simulink model "ext_mode_intro"  (R2017b)
settings: Solver=FixedStepDiscrete  StartTime=0.0  StopTime=inf  FixedStep=1/100  RelTol=1e-3  EnableMultiTasking=on
InitFcn:
  | GainTune = 1;
  | alignTime = floor(398.001 * Ts);
  | EAS2TAS = 1;
  | LatDegInit = 1;
  | LngDegInit = 1;
  | msecVelDelay = 300;
  | msecPosDelay = 300;
  | msecHgtDelay = 420;
  | msecMagDelay = 30;
  | msecTasDelay = 200;
libraries: simulink x9, pixhawk_slib_sensors_actuators x3, simulink_need_slupdate x2
(part 1 of 4)
Description:
  | ext_mode_intro
  | 
  | This model uses ttyS6 on the Pixhawk for the EXT mode serial data exchange.
  | This means the MEX arguments must be set accordingly to use the right COM port.
  | Please check your windows setting (COM8 in this example)
  | COM 6 will be the serial console (ttyACM0)
  | 
  | Note: Baud rate set at 115200
settings Model: SimulationMode=external  Creator=skuznick  LastModifiedBy=tom
settings DataIOCC: LimitDataPoints=on  SaveFormat=Array  SignalLoggingSaveFormat=ModelDataLogs
settings OptimizationCC: DefaultParameterBehavior=Inlined  LifeSpan=1  MaxStackSize=64
settings DebuggingCC: SolverPrmCheckMsg=warning  MultiTaskDSMMsg=warning  MultiTaskCondExecSysMsg=none  AllowSymbolicDim=off  SFUnexpectedBacktrackingDiag=warning  SFNoUnconditionalDefaultTransitionDiag=warning  SFExecutionAtInitializationDiag=none
settings HardwareCC: ProdBitPerPointer=32  ProdBitPerSizeT=32  ProdBitPerPtrDiffT=32  ProdLargestAtomicInteger=Long  ProdLargestAtomicFloat=Double  ProdIntDivRoundTo=Undefined  ProdWordSize=32  ProdHWDeviceType=ARM Compatible->ARM Cortex
settings ModelReferenceCC: PropagateSignalLabelsOutOfModel=off
settings SFSimCC: MATLABDynamicMemAlloc=off
settings RTWCC: SystemTargetFile=ert.tlc  HardwareBoard=Pixhawk PX4  TLCOptions=-aInlineSetEventsForThisBaseRateFcn=TLC_FALSE -aSuppressMultiTaskScheduler=TLC_FALSE -aRateBasedStepFcn=0  TemplateMakefile=ert_default_tmf  GenerateReport=on  Toolchain=Pixhawk Toolchain  IncludeHyperlinkInReport=on  LaunchReport=on  GenerateTraceInfo=on  GenerateTraceReport=on  GenerateTraceReportSl=on  GenerateTraceReportSf=on  GenerateTraceReportEml=on  GenerateCodeMetricsReport=on
settings CodeAppCC: IgnoreCustomStorageClasses=off  StateflowObjectComments=on
settings ERTTargetCC: MultiwordLength=2048  ExtMode=on  ExtModeTransport=1  ExtModeStaticAllocSize=10000  ExtModeMexFile=ext_serial_win32_comm  ExtModeMexArgs=1 '/dev/ttyACM0' 57600 5  ERTCustomFileTemplate=px4_codertarget_file_process.tlc  ConvertIfToSwitch=off  SuppressUnreachableDefaultCases=off
settings ConfigComp: CovMetricSettings=dw  CovHtmlReporting=on  CovSaveCumulativeToWorkspaceVar=on  CovSaveSingleToWorkspaceVar=on  CovExternalEMLEnable=off  CovSFcnEnable=off

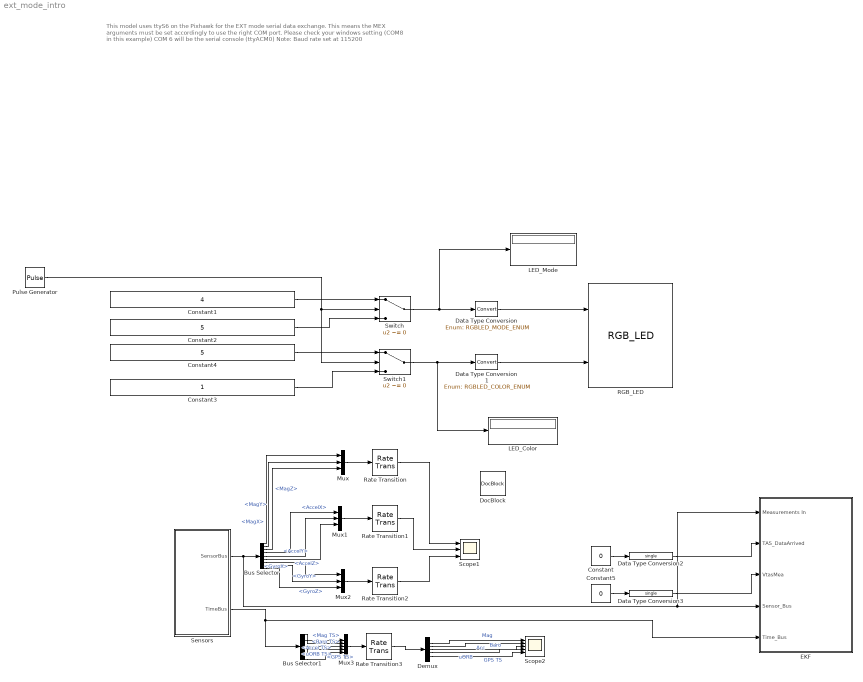
== system ext_mode_intro ==
  note: This model uses ttyS6 on the Pixhawk for the EXT mode serial data exchange.
      | This means the MEX arguments must be set accordingly to use the right COM port.
      | Please check your windows setting (COM8 in this example)
      | COM 6 will be the serial console (ttyACM0)
      |
      | Note: Baud rate set at 115200
  Bus Selector : BusSelector  OutputSignals=MagX,MagY,MagZ,AccelX,AccelY,AccelZ,GyroX,GyroY,GyroZ
  Bus Selector1 : BusSelector  OutputSignals=Mag TS,Accel TS,Baro TS,uORB TS,GPS TS
  Constant : Constant  Value=0  SampleTime=-1
  Constant1 : Constant  Value=4  OutDataTypeStr=int8
  Constant2 : Constant  Value=5  OutDataTypeStr=int8
  Constant3 : Constant  OutDataTypeStr=int8
  Constant4 : Constant  Value=5  OutDataTypeStr=int8
  Constant5 : Constant  Value=0  SampleTime=-1
  Data Type Conversion : DataTypeConversion  OutDataTypeStr=Enum: RGBLED_MODE_ENUM
  Data Type Conversion1 : DataTypeConversion  OutDataTypeStr=Enum: RGBLED_COLOR_ENUM
  Data Type Conversion2 : DataTypeConversion  OutDataTypeStr=single
  Data Type Conversion3 : DataTypeConversion  OutDataTypeStr=single
  Demux : Demux  Outputs=5
  DocBlock : simulink/Model-Wide Utilities/DocBlock  DocumentType=Text
      content=|
      | 24 State Extended Kalman Filter
      |
      | States :
      | 1 ... 4   : Quaternion parameters defining the rotation from local NED tangent frame to XYZ body axes
      | 5 ... 7   : North, East, Down velocity relative to and earth fixed reference point (m)
      | 8 ... 10  : North, East, Down position relative to and earth fixed reference point (m)
      | 11 ... 13 : IMU delta angle bias errors (rad)
      | 14 ... 16 : IMU delta velocity bias errors (m/s)
      | 17,18     : North, East wind velocity (m/s)
      | 19 ... 21 : North, East, Down earth magnetic field (same units as magnetometer output)
      | 22 ... 24 : X, Y, Z Body fixed magnetic field bias - opposite sign to APM offsets (same units as magnetometer output)
      |
      | Time Varying Parameters :
      | IMU delta angles (rad)
      | IMU delta velocity (rad)
      |
      | Observations :
      | North, East, Down velocity (m/s)
      | North, East position (m)
      | Height (m)
      | True Airspeed (m/s) - optional
      | X, Y, Z body fixed magnetic flux measurements (same units as magnetometer output) - optional
      |
      | Note : without compass/magnetometer measurements, the heading alignment cannot be maintained on the ground, so the filter will need to be re-started when flight commences.
      |
      |
      | TO-DO:
      | 1).  Set all signals into a Bus object for cleaner Simulink models.
      | 2).  Incorporate a Complementary filter in the watchdog.
      | 3).  Evaluate EKF model, specificly frequency and parameters.
      | 4).  Tune EKF, Complementary Filter, and controllers for easy angular flight.
      | 5).  Test if all signals are properly connected to the EKF (signs, formats, and representation).
      | 6).  TAS data.
      | 7).  GPS Velocity data.
      | 8).  Include Current measurements to compensate magnetometer.
      | 9).  Include Barometer measurements in EKF.
      | 10). Find out how the reset funtion operates.
  EKF : Subsystem
  LED_Color : Display
  LED_Mode : Display
  Mux : Mux  Inputs=3
  Mux1 : Mux  Inputs=3
  Mux2 : Mux  Inputs=3
  Mux3 : Mux  Inputs=5
  Pulse Generator : DiscretePulseGenerator  PulseType=Time based  Period=6  PulseWidth=50
  RGB_LED : pixhawk_slib_sensors_actuators/RGB_LED
      settings: SourceProductName=Pixhawk Target Blocks
  Rate Transition : RateTransition  InitialCondition=[0; 0; 0]  OutPortSampleTime=0.1
  Rate Transition1 : RateTransition  InitialCondition=[0; 0; 0]  OutPortSampleTime=0.1
  Rate Transition2 : RateTransition  InitialCondition=[0; 0; 0]  OutPortSampleTime=0.1
  Rate Transition3 : RateTransition  InitialCondition=[0; 0; 0; 0; 0]  OutPortSampleTime=0.1
  Scope1 : Scope  NumInputPorts=3
  Scope2 : Scope  NumInputPorts=5
  "Sensors " : Subsystem
  Switch : Switch  Criteria=u2 ~= 0  Threshold=1500
  Switch1 : Switch  Criteria=u2 ~= 0  Threshold=1500
  wires:
  Switch/1 -> LED_Mode/1, Data Type Conversion/1
  Switch1/1 -> LED_Color/1, Data Type Conversion1/1
  Constant1/1 -> Switch/1
  Constant2/1 -> Switch/3
  Constant4/1 -> Switch1/1
  Constant3/1 -> Switch1/3
  Pulse Generator/1 -> Switch1/2, Switch/2
  Data Type Conversion/1 -> RGB_LED/1
  Data Type Conversion1/1 -> RGB_LED/2
  Bus Selector/3 -> Mux/3  "<MagZ>"
  Bus Selector/2 -> Mux/2  "<MagY>"
  Bus Selector/1 -> Mux/1  "<MagX>"
  Bus Selector/6 -> Mux1/3  "<AccelZ>"
  Bus Selector/5 -> Mux1/2  "<AccelY>"
  Bus Selector/4 -> Mux1/1  "<AccelX>"
  Bus Selector/7 -> Mux2/1  "<GyroX>"
  Bus Selector/8 -> Mux2/2  "<GyroY>"
  Bus Selector/9 -> Mux2/3  "<GyroZ>"
  Mux/1 -> Rate Transition/1
  Mux1/1 -> Rate Transition1/1
  Mux2/1 -> Rate Transition2/1
  Rate Transition/1 -> Scope1/1
  Rate Transition1/1 -> Scope1/2
  Rate Transition2/1 -> Scope1/3
  Constant/1 -> Data Type Conversion2/1
  Data Type Conversion2/1 -> EKF/2(TAS_DataArrived)
  Constant5/1 -> Data Type Conversion3/1
  Data Type Conversion3/1 -> EKF/3(VtasMea)
  "Sensors "/1(SensorBus) -> EKF/4(Sensor_Bus), EKF/1(Measurements In), Bus Selector/1
  Bus Selector1/1 -> Mux3/1  "<Mag TS>"
  Bus Selector1/2 -> Mux3/2  "<Accel TS>"
  Bus Selector1/3 -> Mux3/3  "<Baro TS>"
  Bus Selector1/4 -> Mux3/4  "<uORB TS>"
  Mux3/1 -> Rate Transition3/1
  Rate Transition3/1 -> Demux/1
  Demux/1 -> Scope2/1  "Mag"
  Demux/2 -> Scope2/2  "Acc"
  Demux/3 -> Scope2/3  "Baro"
  Demux/4 -> Scope2/4  "uORB"
  "Sensors "/2(TimeBus) -> EKF/5(Time_Bus), Bus Selector1/1
  Bus Selector1/5 -> Mux3/5  "<GPS TS>"
  Demux/5 -> Scope2/5  "GPS TS"

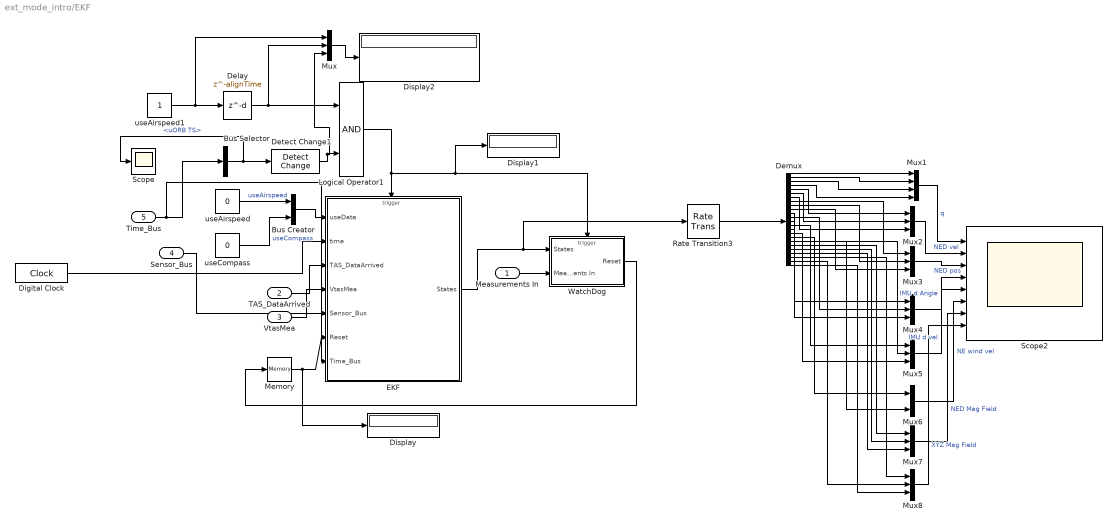
== system ext_mode_intro/EKF ==
  Measurements In : Inport
  TAS_DataArrived : Inport  Port=2
  VtasMea : Inport  Port=3
  Sensor_Bus : Inport  Port=4
  Time_Bus : Inport  Port=5
  Bus Creator : BusCreator  Inputs=2
  Bus Selector : BusSelector  OutputSignals=uORB TS
  Delay : Delay  DelayLength=alignTime  InitialCondition=0
  Demux : Demux  Outputs=24
  Detect Change1 : simulink/Logic and Bit Operations/Detect Change  vinit=0  InputProcessing=Inherited  OutDataTypeStr=boolean
  Digital Clock : DigitalClock  SampleTime=-1
  Display : Display
  Display1 : Display
  Display2 : Display
  EKF : Subsystem
  Logical Operator1 : Logic  AllPortsSameDT=off  OutDataTypeStr=boolean
  Memory : Memory  InheritSampleTime=on
  Mux{,2..5,7..8} (7 alike) : Mux  Inputs=3
  Mux1 : Mux
  Mux6 : Mux  Inputs=2
  Rate Transition3 : RateTransition  InitialCondition=zeros(24,1)  OutPortSampleTime=0.1
  Scope : Scope
  Scope2 : Scope  NumInputPorts=8
  WatchDog : Subsystem  TreatAsAtomicUnit=on
  useAirspeed : Constant  Value=0  OutDataTypeStr=boolean  SampleTime=-1
  useAirspeed1 : Constant  OutDataTypeStr=boolean  SampleTime=-1
  useCompass : Constant  Value=0  OutDataTypeStr=boolean  SampleTime=-1
  wires:
  Measurements In/1 -> WatchDog/2(Measurements In)
  useAirspeed/1 -> Bus Creator/1  "useAirspeed"
  useCompass/1 -> Bus Creator/2  "useCompass"
  EKF/1(States) -> Rate Transition3/1, WatchDog/1(States)
  Logical Operator1/1 -> Display1/1, WatchDog/Trigger, EKF/Trigger
  Memory/1 -> Display/1, EKF/6(Reset)
  WatchDog/1(Reset) -> Memory/1
  Detect Change1/1 -> Mux/3, Logical Operator1/2
  Delay/1 -> Mux/2, Logical Operator1/1
  TAS_DataArrived/1 -> EKF/3(TAS_DataArrived)
  VtasMea/1 -> EKF/4(VtasMea)
  Sensor_Bus/1 -> EKF/5(Sensor_Bus)
  Bus Selector/1 -> Scope/1, Detect Change1/1  "<uORB TS>"
  Bus Creator/1 -> EKF/1(useData)
  useAirspeed1/1 -> Mux/1, Delay/1
  Digital Clock/1 -> EKF/2(time)
  Mux/1 -> Display2/1
  Time_Bus/1 -> EKF/7(Time_Bus), Bus Selector/1
  Rate Transition3/1 -> Demux/1
  Demux/1 -> Mux1/1
  Demux/2 -> Mux1/2
  Demux/3 -> Mux1/3
  Demux/4 -> Mux1/4
  Mux1/1 -> Scope2/1  "q"
  Demux/5 -> Mux2/1
  Demux/6 -> Mux2/2
  Demux/7 -> Mux2/3
  Mux2/1 -> Scope2/2  "NED vel"
  Demux/8 -> Mux3/1
  Demux/9 -> Mux3/2
  Demux/10 -> Mux3/3
  Mux3/1 -> Scope2/3  "NED pos"
  Demux/11 -> Mux4/1
  Demux/12 -> Mux4/2
  Demux/13 -> Mux4/3
  Mux4/1 -> Scope2/4  "IMU d Angle"
  Demux/14 -> Mux5/1
  Demux/15 -> Mux5/2
  Demux/16 -> Mux5/3
  Mux5/1 -> Scope2/5  "IMU d vel"
  Demux/17 -> Mux6/1
  Demux/18 -> Mux6/2
  Mux6/1 -> Scope2/6  "NE wind vel"
  Demux/19 -> Mux7/1
  Demux/20 -> Mux7/2
  Demux/21 -> Mux7/3
  Demux/22 -> Mux8/1
  Demux/23 -> Mux8/2
  Demux/24 -> Mux8/3
  Mux7/1 -> Scope2/7  "NED Mag Field"
  Mux8/1 -> Scope2/8  "XYZ Mag Field"

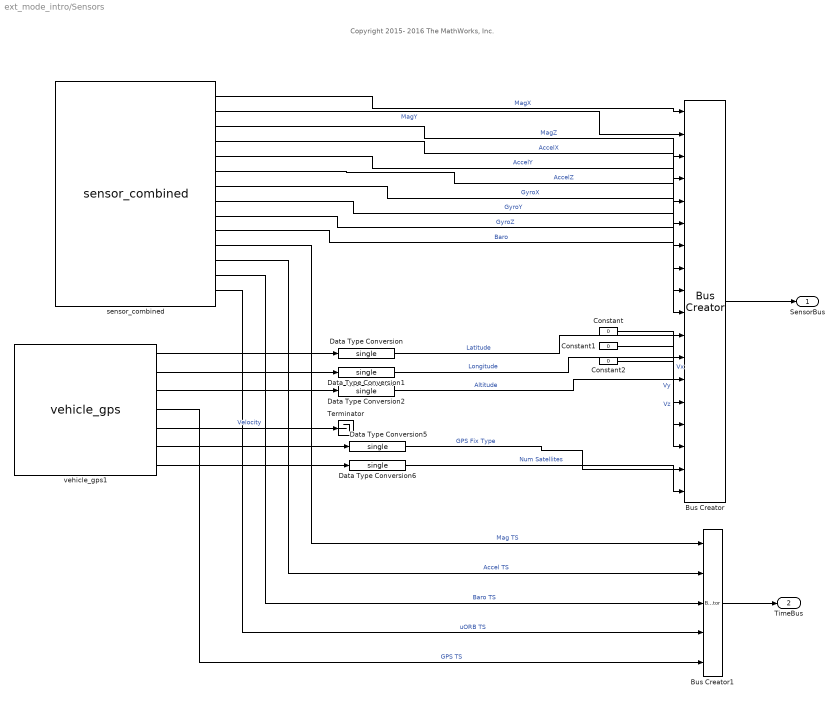
== system ext_mode_intro/Sensors  ==
  note: Copyright 2015- 2016 The MathWorks, Inc.
  Bus Creator : BusCreator  Inputs=18
  Bus Creator1 : BusCreator  Inputs=5
  Constant : Constant  Value=0  OutDataTypeStr=single  SampleTime=-1
  Constant1 : Constant  Value=0  OutDataTypeStr=single  SampleTime=-1
  Constant2 : Constant  Value=0  OutDataTypeStr=single  SampleTime=-1
  Data Type Conversion{,1..2,5..6} (5 alike) : DataTypeConversion  OutDataTypeStr=single
  Terminator : Terminator
  sensor_combined : pixhawk_slib_sensors_actuators/sensor_combined  Description=|  sampletime=-1  show_mag=on  show_acc=on  show_gyro=on  show_baro=on  show_ts=on
      | Sensor Combined Block
      | 
      | This block enables access to the various sensors available on the px4fmu-v2 hardware.  
      | The user can use these signals in the Simulink control model.  
      | The sample time needs to be provided in the mask dialog.  
      | Optional output ports can also be selected.  
      | Refer to the sample model: px4demo_attitude_control.slx
      | 
      | Signal definitions: 
      | Magnetometer (x,y,z) - single values – Magnetic field in NED body frame, in Gauss 
      | Accelerometer (x,y,z) - single values – Acceleration in NED body frame, in m/s^2 
      | Gyroscope (p,q,r) - single values – Angular velocity in radians per second 
      | Barometer (Altitude) - single value – Barometric pressure, already temperature compensated (millibars) 
      | RunTime (timestamp) - double value – Timestamp in microseconds since boot, from gyro 
      |   
      | The sensor_combined block needs to have the px4io service running on the PX4 hardware in order to get valid signal values.
      settings: SourceProductName=Pixhawk Target Blocks
  vehicle_gps1 : pixhawk_slib_sensors_actuators/vehicle_gps  sampletime=-1  show_alt=on  show_ts_gps=on  show_vel=on  show_fixtype=on  show_numsat=on
      settings: SourceProductName=Pixhawk Target Blocks
  SensorBus : Outport
  TimeBus : Outport  Port=2
  wires:
  sensor_combined/1 -> Bus Creator/1  "MagX"
  sensor_combined/2 -> Bus Creator/2  "MagY"
  sensor_combined/3 -> Bus Creator/3  "MagZ"
  sensor_combined/7 -> Bus Creator/7  "GyroX"
  sensor_combined/8 -> Bus Creator/8  "GyroY"
  sensor_combined/9 -> Bus Creator/9  "GyroZ"
  sensor_combined/4 -> Bus Creator/4  "AccelX"
  sensor_combined/5 -> Bus Creator/5  "AccelY"
  sensor_combined/6 -> Bus Creator/6  "AccelZ"
  sensor_combined/10 -> Bus Creator/10  "Baro"
  vehicle_gps1/1 -> Data Type Conversion/1
  vehicle_gps1/2 -> Data Type Conversion1/1
  vehicle_gps1/3 -> Data Type Conversion2/1
  vehicle_gps1/6 -> Data Type Conversion5/1
  vehicle_gps1/7 -> Data Type Conversion6/1
  Bus Creator/1 -> SensorBus/1
  vehicle_gps1/5 -> Terminator/1  "Velocity"
  Data Type Conversion/1 -> Bus Creator/11  "Latitude"
  Data Type Conversion1/1 -> Bus Creator/12  "Longitude"
  Data Type Conversion2/1 -> Bus Creator/13  "Altitude"
  Data Type Conversion5/1 -> Bus Creator/17  "GPS Fix Type"
  Data Type Conversion6/1 -> Bus Creator/18  "Num Satellites"
  Constant/1 -> Bus Creator/14  "Vx"
  Constant1/1 -> Bus Creator/15  "Vy"
  Constant2/1 -> Bus Creator/16  "Vz"
  sensor_combined/14 -> Bus Creator1/4  "uORB TS"
  sensor_combined/13 -> Bus Creator1/3  "Baro TS"
  sensor_combined/12 -> Bus Creator1/2  "Accel TS"
  sensor_combined/11 -> Bus Creator1/1  "Mag TS"
  vehicle_gps1/4 -> Bus Creator1/5  "GPS TS"
  Bus Creator1/1 -> TimeBus/1

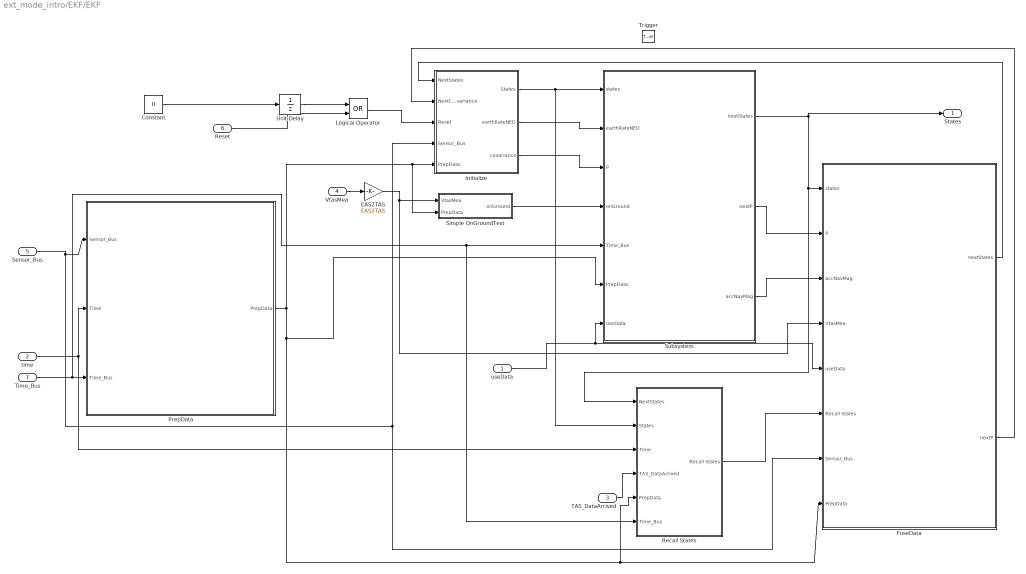
== system ext_mode_intro/EKF/EKF ==
  useData : Inport  OutDataTypeStr=boolean
  time : Inport  Port=2  OutDataTypeStr=double  PortDimensions=1
  TAS_DataArrived : Inport  Port=3
  VtasMea : Inport  Port=4
  Sensor_Bus : Inport  Port=5
  Reset : Inport  Port=6  OutDataTypeStr=boolean  PortDimensions=1
  Time_Bus : Inport  Port=7  OutDataTypeStr=double
  Trigger : TriggerPort  VariantControl=(inherit)  PortDimensions=1
  Constant : Constant  Value=0  OutDataTypeStr=boolean  SampleTime=-1
  EAS2TAS : Gain  Gain=EAS2TAS
  FuseData : Subsystem
  Initialize : Subsystem
  Logical Operator : Logic  Operator=OR  AllPortsSameDT=off  OutDataTypeStr=boolean
  PrepData : Subsystem
  Recall States : Subsystem
  Simple OnGroundTest : Subsystem  TreatAsAtomicUnit=on
  Subsystem : Subsystem
  Unit Delay : UnitDelay  InitialCondition=1  SampleTime=-1
  States : Outport  OutDataTypeStr=single  PortDimensions=24
  wires:
  time/1 -> Recall States/3(Time), PrepData/2(Time)
  Unit Delay/1 -> Logical Operator/1
  Logical Operator/1 -> Initialize/3(Reset)
  Initialize/1(States) -> Subsystem/1(states), Recall States/2(States)
  Reset/1 -> Logical Operator/2
  VtasMea/1 -> EAS2TAS/1
  Sensor_Bus/1 -> PrepData/1(Sensor_Bus), FuseData/7(Sensor_Bus), Initialize/4(Sensor_Bus)
  Constant/1 -> Unit Delay/1
  EAS2TAS/1 -> FuseData/4(VtasMea), Simple OnGroundTest/1(VtasMea)
  Subsystem/1(nextStates) -> States/1, Recall States/1(NextStates), FuseData/1(states)
  Initialize/2(earthRateNED) -> Subsystem/2(earthRateNED)
  Initialize/3(covariance) -> Subsystem/3(P)
  Simple OnGroundTest/1(onGround) -> Subsystem/4(onGround)
  Subsystem/2(nextP) -> FuseData/2(P)
  Subsystem/3(accNavMag) -> FuseData/3(accNavMag)
  FuseData/1(nextStates) -> Initialize/1(NextStates)
  FuseData/2(nextP) -> Initialize/2(NextCovariance)
  TAS_DataArrived/1 -> Recall States/4(TAS_DataArrived)
  useData/1 -> Subsystem/7(useData), FuseData/5(useData)
  Recall States/1(Recall States) -> FuseData/6(Recall States)
  PrepData/1(PrepData) -> Recall States/5(PrepData), FuseData/8(PrepData), Subsystem/6(PrepData), Simple OnGroundTest/2(PrepData), Initialize/5(PrepData)
  Time_Bus/1 -> Recall States/6(Time_Bus), Subsystem/5(Time_Bus), PrepData/3(Time_Bus)

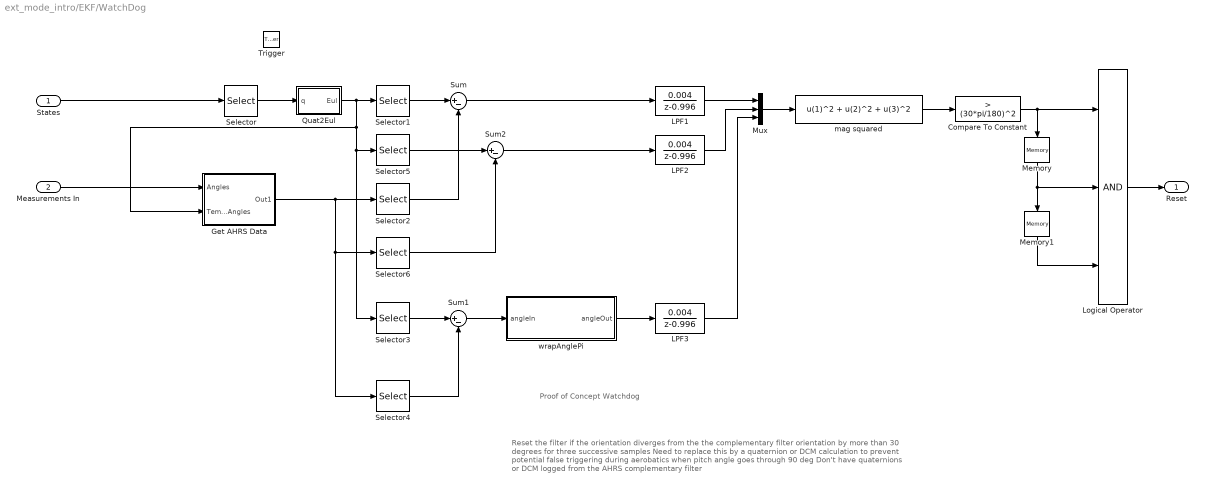
== system ext_mode_intro/EKF/WatchDog ==
  note: Reset the filter if the orientation diverges from the the complementary filter orientation  by more than 30 degrees for three successive samples
      | Need to replace this by a quaternion or DCM calculation to prevent potential false triggering during aerobatics when pitch angle goes through 90 deg
      | Don't have quaternions or DCM logged from the AHRS complementary filter
  note: Proof of Concept Watchdog
  States : Inport
  Measurements In : Inport  Port=2
  Trigger : TriggerPort  VariantControl=(inherit)  PortDimensions=1
  Compare To Constant : simulink/Logic and Bit Operations/Compare To Constant  relop=>  const=(30*pi/180)^2  OutDataTypeStr=boolean
  Get AHRS Data : Subsystem
  LPF1 : DiscreteTransferFcn  Numerator=0.004  Denominator=[1 -0.996]
  LPF2 : DiscreteTransferFcn  Numerator=0.004  Denominator=[1 -0.996]
  LPF3 : DiscreteTransferFcn  Numerator=0.004  Denominator=[1 -0.996]
  Logical Operator : Logic  Inputs=3  AllPortsSameDT=off  OutDataTypeStr=boolean
  Memory : Memory  InheritSampleTime=on
  Memory1 : Memory  InheritSampleTime=on
  Mux : Mux  Inputs=3
  Quat2Eul : Subsystem
  Selector : Selector  InputPortWidth=24  IndexOptions=Index vector (dialog)  Indices=[1:4]  OutputSizes=1
  Selector1 : Selector  InputPortWidth=3  IndexOptions=Index vector (dialog)  Indices=1  OutputSizes=1
  Selector2 : Selector  InputPortWidth=3  IndexOptions=Index vector (dialog)  Indices=1  OutputSizes=1
  Selector3 : Selector  InputPortWidth=3  IndexOptions=Index vector (dialog)  Indices=3  OutputSizes=1
  Selector4 : Selector  InputPortWidth=3  IndexOptions=Index vector (dialog)  Indices=3  OutputSizes=1
  Selector5 : Selector  InputPortWidth=3  IndexOptions=Index vector (dialog)  Indices=2  OutputSizes=1
  Selector6 : Selector  InputPortWidth=3  IndexOptions=Index vector (dialog)  Indices=2  OutputSizes=1
  Sum : Sum  Inputs=|+-
  Sum1 : Sum  Inputs=|+-
  Sum2 : Sum  Inputs=|+-
  mag squared : Fcn  Expr=u(1)^2 + u(2)^2 + u(3)^2
  wrapAnglePi : MATLAB Function  TreatAsAtomicUnit=on
  Reset : Outport  OutDataTypeStr=boolean  PortDimensions=1
  wires:
  Selector/1 -> Quat2Eul/1(q)
  States/1 -> Selector/1
  Quat2Eul/1(Eul) -> Selector1/1, Get AHRS Data/2(Temp Angles), Selector3/1, Selector5/1
  Get AHRS Data/1(Out1) -> Selector2/1, Selector4/1, Selector6/1
  Selector3/1 -> Sum1/1
  Selector4/1 -> Sum1/2
  Sum1/1 -> wrapAnglePi/1(angleIn)
  Sum/1 -> LPF1/1
  wrapAnglePi/1(angleOut) -> LPF3/1
  Mux/1 -> mag squared/1
  mag squared/1 -> Compare To Constant/1
  Compare To Constant/1 -> Logical Operator/1, Memory/1
  Logical Operator/1 -> Reset/1
  Memory/1 -> Logical Operator/2, Memory1/1
  Memory1/1 -> Logical Operator/3
  Selector1/1 -> Sum/1
  Selector2/1 -> Sum/2
  Selector5/1 -> Sum2/1
  Selector6/1 -> Sum2/2
  Sum2/1 -> LPF2/1
  LPF1/1 -> Mux/1
  LPF2/1 -> Mux/2
  LPF3/1 -> Mux/3
  Measurements In/1 -> Get AHRS Data/1(Angles)

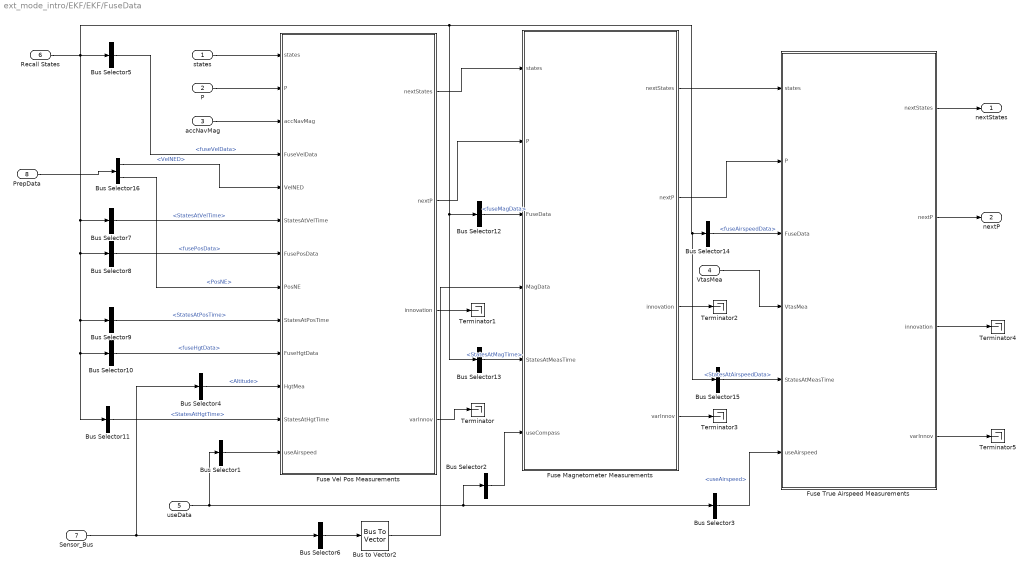
== system ext_mode_intro/EKF/EKF/FuseData ==
  states : Inport
  P : Inport  Port=2
  accNavMag : Inport  Port=3
  VtasMea : Inport  Port=4
  useData : Inport  Port=5
  Recall States : Inport  Port=6
  Sensor_Bus : Inport  Port=7
  PrepData : Inport  Port=8
  Bus Selector1 : BusSelector  OutputSignals=useAirspeed  OutputAsBus=on
  Bus Selector10 : BusSelector  OutputSignals=fuseHgtData
  Bus Selector11 : BusSelector  OutputSignals=StatesAtHgtTime
  Bus Selector12 : BusSelector  OutputSignals=fuseMagData
  Bus Selector13 : BusSelector  OutputSignals=StatesAtMagTime
  Bus Selector14 : BusSelector  OutputSignals=fuseAirspeedData
  Bus Selector15 : BusSelector  OutputSignals=StatesAtAirspeedData
  Bus Selector16 : BusSelector  OutputSignals=VelNED,PosNE
  Bus Selector2 : BusSelector  OutputSignals=useCompass  OutputAsBus=on
  Bus Selector3 : BusSelector  OutputSignals=useAirspeed
  Bus Selector4 : BusSelector  OutputSignals=Altitude
  Bus Selector5 : BusSelector  OutputSignals=fuseVelData
  Bus Selector6 : BusSelector  OutputSignals=MagX,MagY,MagZ  OutputAsBus=on
  Bus Selector7 : BusSelector  OutputSignals=StatesAtVelTime
  Bus Selector8 : BusSelector  OutputSignals=fusePosData
  Bus Selector9 : BusSelector  OutputSignals=StatesAtPosTime
  Bus to Vector2 : BusToVector
  Fuse Magnetometer Measurements : MATLAB Function  TreatAsAtomicUnit=on
  Fuse True Airspeed Measurements : MATLAB Function  TreatAsAtomicUnit=on
  Fuse Vel Pos Measurements : MATLAB Function  TreatAsAtomicUnit=on
  Terminator{,1..5} (6 alike) : Terminator
  nextStates : Outport
  nextP : Outport  Port=2
  wires:
  Bus Selector2/1 -> Fuse Magnetometer Measurements/6(useCompass)
  accNavMag/1 -> Fuse Vel Pos Measurements/3(accNavMag)
  Bus Selector16/1 -> Fuse Vel Pos Measurements/5(VelNED)  "<VelNED>"
  Bus Selector16/2 -> Fuse Vel Pos Measurements/8(PosNE)  "<PosNE>"
  VtasMea/1 -> Fuse True Airspeed Measurements/4(VtasMea)
  Bus Selector1/1 -> Fuse Vel Pos Measurements/13(useAirspeed)
  states/1 -> Fuse Vel Pos Measurements/1(states)
  Bus to Vector2/1 -> Fuse Magnetometer Measurements/4(MagData)
  Fuse Vel Pos Measurements/2(nextP) -> Fuse Magnetometer Measurements/2(P)
  Bus Selector4/1 -> Fuse Vel Pos Measurements/11(HgtMea)  "<Altitude>"
  Fuse Magnetometer Measurements/2(nextP) -> Fuse True Airspeed Measurements/2(P)
  Bus Selector8/1 -> Fuse Vel Pos Measurements/7(FusePosData)  "<fusePosData>"
  Bus Selector5/1 -> Fuse Vel Pos Measurements/4(FuseVelData)  "<fuseVelData>"
  Bus Selector13/1 -> Fuse Magnetometer Measurements/5(StatesAtMeasTime)  "<StatesAtMagTime>"
  Bus Selector7/1 -> Fuse Vel Pos Measurements/6(StatesAtVelTime)  "<StatesAtVelTime>"
  Bus Selector12/1 -> Fuse Magnetometer Measurements/3(FuseData)  "<fuseMagData>"
  Recall States/1 -> Bus Selector13/1, Bus Selector12/1, Bus Selector15/1, Bus Selector14/1, Bus Selector11/1, Bus Selector10/1, Bus Selector9/1, Bus Selector8/1, Bus Selector7/1, Bus Selector5/1
  Bus Selector10/1 -> Fuse Vel Pos Measurements/10(FuseHgtData)  "<fuseHgtData>"
  Fuse Vel Pos Measurements/1(nextStates) -> Fuse Magnetometer Measurements/1(states)
  Fuse True Airspeed Measurements/1(nextStates) -> nextStates/1
  Bus Selector9/1 -> Fuse Vel Pos Measurements/9(StatesAtPosTime)  "<StatesAtPosTime>"
  Fuse True Airspeed Measurements/2(nextP) -> nextP/1
  Fuse Magnetometer Measurements/1(nextStates) -> Fuse True Airspeed Measurements/1(states)
  Bus Selector11/1 -> Fuse Vel Pos Measurements/12(StatesAtHgtTime)  "<StatesAtHgtTime>"
  Bus Selector15/1 -> Fuse True Airspeed Measurements/5(StatesAtMeasTime)  "<StatesAtAirspeedData>"
  Fuse Vel Pos Measurements/3(innovation) -> Terminator1/1
  Fuse Vel Pos Measurements/4(varInnov) -> Terminator/1
  Fuse Magnetometer Measurements/3(innovation) -> Terminator2/1
  Fuse Magnetometer Measurements/4(varInnov) -> Terminator3/1
  Fuse True Airspeed Measurements/3(innovation) -> Terminator4/1
  P/1 -> Fuse Vel Pos Measurements/2(P)
  Fuse True Airspeed Measurements/4(varInnov) -> Terminator5/1
  Bus Selector6/1 -> Bus to Vector2/1
  useData/1 -> Bus Selector1/1, Bus Selector2/1, Bus Selector3/1
  Bus Selector3/1 -> Fuse True Airspeed Measurements/6(useAirspeed)  "<useAirspeed>"
  Sensor_Bus/1 -> Bus Selector6/1, Bus Selector4/1
  Bus Selector14/1 -> Fuse True Airspeed Measurements/3(FuseData)  "<fuseAirspeedData>"
  PrepData/1 -> Bus Selector16/1

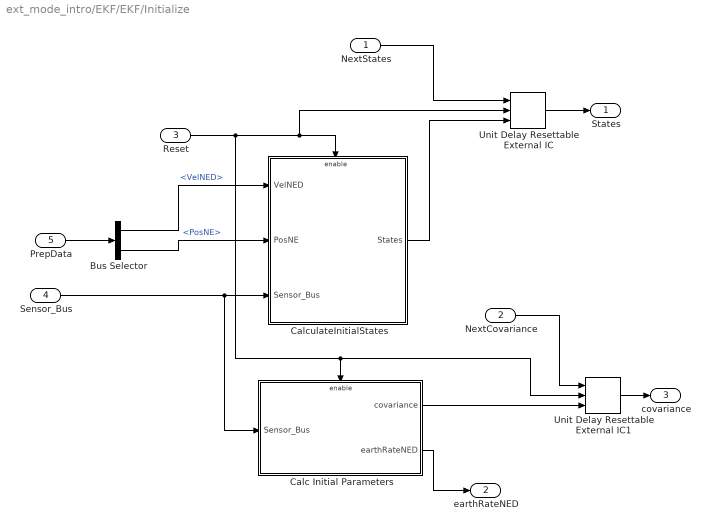
== system ext_mode_intro/EKF/EKF/Initialize ==
  NextStates : Inport
  NextCovariance : Inport  Port=2
  Reset : Inport  Port=3
  Sensor_Bus : Inport  Port=4
  PrepData : Inport  Port=5
  Bus Selector : BusSelector  OutputSignals=VelNED,PosNE
  Calc Initial Parameters : Subsystem
  CalculateInitialStates : Subsystem  TreatAsAtomicUnit=on
  Unit Delay Resettable External IC : simulink_need_slupdate/Unit Delay Resettable External IC  tsamp=-1
      settings: SourceProductName=Simulink  SourceProductBaseCode=SL
  Unit Delay Resettable External IC1 : simulink_need_slupdate/Unit Delay Resettable External IC  tsamp=-1
      settings: SourceProductName=Simulink  SourceProductBaseCode=SL
  States : Outport
  earthRateNED : Outport  Port=2
  covariance : Outport  Port=3
  wires:
  Sensor_Bus/1 -> Calc Initial Parameters/1(Sensor_Bus), CalculateInitialStates/3(Sensor_Bus)
  Bus Selector/1 -> CalculateInitialStates/1(VelNED)  "<VelNED>"
  Reset/1 -> Unit Delay Resettable External IC1/2, Calc Initial Parameters/Enable, Unit Delay Resettable External IC/2, CalculateInitialStates/Enable
  Bus Selector/2 -> CalculateInitialStates/2(PosNE)  "<PosNE>"
  CalculateInitialStates/1(States) -> Unit Delay Resettable External IC/3
  Unit Delay Resettable External IC/1 -> States/1
  NextStates/1 -> Unit Delay Resettable External IC/1
  Calc Initial Parameters/2(earthRateNED) -> earthRateNED/1
  Calc Initial Parameters/1(covariance) -> Unit Delay Resettable External IC1/3
  NextCovariance/1 -> Unit Delay Resettable External IC1/1
  Unit Delay Resettable External IC1/1 -> covariance/1
  PrepData/1 -> Bus Selector/1

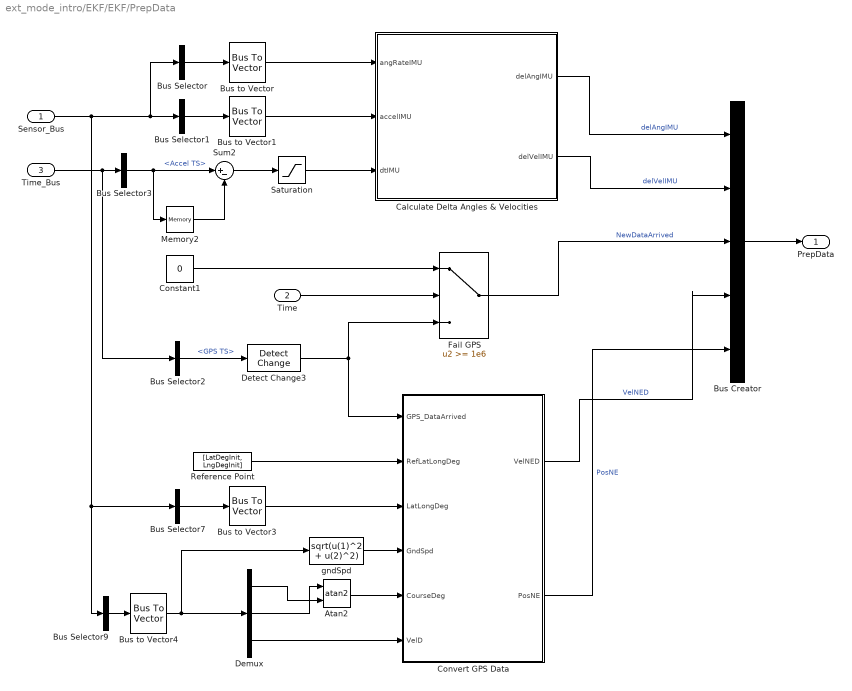
== system ext_mode_intro/EKF/EKF/PrepData ==
  Sensor_Bus : Inport
  Time : Inport  Port=2
  Time_Bus : Inport  Port=3
  Atan2 : Trigonometry  Operator=atan2
  Bus Creator : BusCreator  Inputs=5
  Bus Selector : BusSelector  OutputSignals=GyroX,GyroY,GyroZ  OutputAsBus=on
  Bus Selector1 : BusSelector  OutputSignals=AccelX,AccelY,AccelZ  OutputAsBus=on
  Bus Selector2 : BusSelector  OutputSignals=GPS TS
  Bus Selector3 : BusSelector  OutputSignals=Accel TS
  Bus Selector7 : BusSelector  OutputSignals=Latitude,Longitude  OutputAsBus=on
  Bus Selector9 : BusSelector  OutputSignals=Vx,Vy,Vz  OutputAsBus=on
  Bus to Vector{,1,3..4} (4 alike) : BusToVector
  Calculate Delta Angles & Velocities : MATLAB Function  TreatAsAtomicUnit=on
  Constant1 : Constant  Value=0  OutDataTypeStr=boolean
  Convert GPS Data : MATLAB Function  TreatAsAtomicUnit=on
  Demux : Demux  Outputs=3
  Detect Change3 : simulink/Logic and Bit Operations/Detect Change  vinit=0  InputProcessing=Inherited  OutDataTypeStr=boolean
  Fail GPS : Switch  Threshold=1e6
  Memory2 : Memory  InheritSampleTime=on
  Reference Point : Constant  Value=[LatDegInit, LngDegInit]  OutDataTypeStr=single
  Saturation : Saturate  UpperLimit=0.04  LowerLimit=0
  Sum2 : Sum  Inputs=|+-  AccumDataTypeStr=single
  gndSpd : Fcn  Expr=sqrt(u(1)^2 + u(2)^2)
  PrepData : Outport
  wires:
  Fail GPS/1 -> Bus Creator/3  "NewDataArrived"
  Detect Change3/1 -> Convert GPS Data/1(GPS_DataArrived), Fail GPS/3
  Saturation/1 -> Calculate Delta Angles & Velocities/3(dtIMU)
  Calculate Delta Angles & Velocities/2(delVelIMU) -> Bus Creator/2  "delVelIMU"
  Calculate Delta Angles & Velocities/1(delAngIMU) -> Bus Creator/1  "delAngIMU"
  Convert GPS Data/1(VelNED) -> Bus Creator/4  "VelNED"
  Convert GPS Data/2(PosNE) -> Bus Creator/5  "PosNE"
  Bus to Vector1/1 -> Calculate Delta Angles & Velocities/2(accelIMU)
  Constant1/1 -> Fail GPS/1
  Reference Point/1 -> Convert GPS Data/2(RefLatLongDeg)
  gndSpd/1 -> Convert GPS Data/4(GndSpd)
  Atan2/1 -> Convert GPS Data/5(CourseDeg)
  Demux/3 -> Convert GPS Data/6(VelD)
  Time/1 -> Fail GPS/2
  Bus to Vector3/1 -> Convert GPS Data/3(LatLongDeg)
  Bus Selector/1 -> Bus to Vector/1
  Bus to Vector/1 -> Calculate Delta Angles & Velocities/1(angRateIMU)
  Bus Selector1/1 -> Bus to Vector1/1
  Bus Selector9/1 -> Bus to Vector4/1
  Bus to Vector4/1 -> gndSpd/1, Demux/1
  Demux/1 -> Atan2/2
  Demux/2 -> Atan2/1
  Bus Selector7/1 -> Bus to Vector3/1
  Sensor_Bus/1 -> Bus Selector/1, Bus Selector1/1, Bus Selector7/1, Bus Selector9/1
  Bus Selector2/1 -> Detect Change3/1  "<GPS TS>"
  Memory2/1 -> Sum2/2
  Bus Selector3/1 -> Sum2/1, Memory2/1  "<Accel TS>"
  Sum2/1 -> Saturation/1
  Bus Creator/1 -> PrepData/1
  Time_Bus/1 -> Bus Selector2/1, Bus Selector3/1

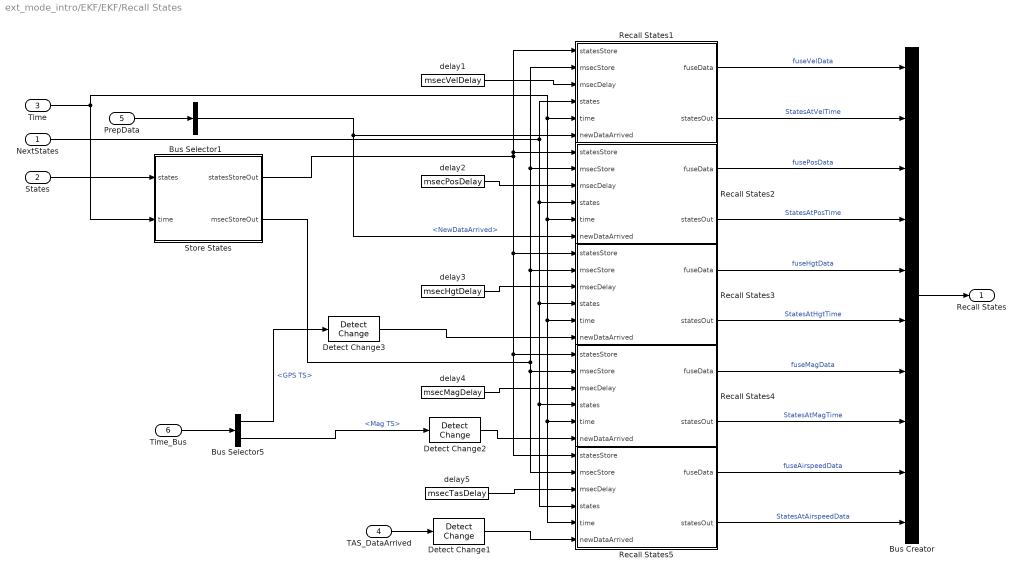
== system ext_mode_intro/EKF/EKF/Recall States ==
  NextStates : Inport
  States : Inport  Port=2
  Time : Inport  Port=3
  TAS_DataArrived : Inport  Port=4
  PrepData : Inport  Port=5
  Time_Bus : Inport  Port=6
  Bus Creator : BusCreator  Inputs=10
  Bus Selector1 : BusSelector  OutputSignals=NewDataArrived
  Bus Selector5 : BusSelector  OutputSignals=GPS TS,Mag TS
  Detect Change1 : simulink/Logic and Bit Operations/Detect Change  vinit=0  InputProcessing=Inherited  OutDataTypeStr=boolean
  Detect Change2 : simulink/Logic and Bit Operations/Detect Change  vinit=0  InputProcessing=Inherited  OutDataTypeStr=boolean
  Detect Change3 : simulink/Logic and Bit Operations/Detect Change  vinit=0  InputProcessing=Inherited  OutDataTypeStr=boolean
  Recall States1 : MATLAB Function  TreatAsAtomicUnit=on
  Recall States2 : MATLAB Function  TreatAsAtomicUnit=on
  Recall States3 : MATLAB Function  TreatAsAtomicUnit=on
  Recall States4 : MATLAB Function  TreatAsAtomicUnit=on
  Recall States5 : MATLAB Function  TreatAsAtomicUnit=on
  Store States : MATLAB Function  TreatAsAtomicUnit=on
  delay1 : Constant  Value=msecVelDelay  OutDataTypeStr=int32  SampleTime=-1
  delay2 : Constant  Value=msecPosDelay  OutDataTypeStr=int32  SampleTime=-1
  delay3 : Constant  Value=msecHgtDelay  OutDataTypeStr=int32  SampleTime=-1
  delay4 : Constant  Value=msecMagDelay  OutDataTypeStr=int32  SampleTime=-1
  delay5 : Constant  Value=msecTasDelay  OutDataTypeStr=int32  SampleTime=-1
  Recall States : Outport
  wires:
  Recall States4/1(fuseData) -> Bus Creator/7  "fuseMagData"
  Recall States5/2(statesOut) -> Bus Creator/10  "StatesAtAirspeedData"
  Recall States1/2(statesOut) -> Bus Creator/2  "StatesAtVelTime"
  Recall States1/1(fuseData) -> Bus Creator/1  "fuseVelData"
  Recall States2/1(fuseData) -> Bus Creator/3  "fusePosData"
  Recall States2/2(statesOut) -> Bus Creator/4  "StatesAtPosTime"
  Recall States4/2(statesOut) -> Bus Creator/8  "StatesAtMagTime"
  NextStates/1 -> Recall States1/4(states), Recall States5/4(states), Recall States4/4(states), Recall States3/4(states), Recall States2/4(states)
  Recall States5/1(fuseData) -> Bus Creator/9  "fuseAirspeedData"
  Recall States3/1(fuseData) -> Bus Creator/5  "fuseHgtData"
  Recall States3/2(statesOut) -> Bus Creator/6  "StatesAtHgtTime"
  delay2/1 -> Recall States2/3(msecDelay)
  delay5/1 -> Recall States5/3(msecDelay)
  Store States/1(statesStoreOut) -> Recall States1/1(statesStore), Recall States2/1(statesStore), Recall States5/1(statesStore), Recall States4/1(statesStore), Recall States3/1(statesStore)
  delay4/1 -> Recall States4/3(msecDelay)
  Detect Change2/1 -> Recall States4/6(newDataArrived)
  Store States/2(msecStoreOut) -> Recall States1/2(msecStore), Recall States2/2(msecStore), Recall States3/2(msecStore), Recall States5/2(msecStore), Recall States4/2(msecStore)
  Bus Selector1/1 -> Recall States2/6(newDataArrived), Recall States1/6(newDataArrived)  "<NewDataArrived>"
  delay1/1 -> Recall States1/3(msecDelay)
  delay3/1 -> Recall States3/3(msecDelay)
  TAS_DataArrived/1 -> Detect Change1/1
  Detect Change3/1 -> Recall States3/6(newDataArrived)
  Detect Change1/1 -> Recall States5/6(newDataArrived)
  Bus Selector5/1 -> Detect Change3/1  "<GPS TS>"
  Bus Selector5/2 -> Detect Change2/1  "<Mag TS>"
  Time/1 -> Store States/2(time), Recall States1/5(time), Recall States3/5(time), Recall States5/5(time), Recall States4/5(time), Recall States2/5(time)
  States/1 -> Store States/1(states)
  Bus Creator/1 -> Recall States/1
  PrepData/1 -> Bus Selector1/1
  Time_Bus/1 -> Bus Selector5/1

== system ext_mode_intro/EKF/EKF/Simple OnGroundTest ==
  VtasMea : Inport
  PrepData : Inport  Port=2
  Bus Selector : BusSelector  OutputSignals=VelNED
  Logical Operator : Logic  AllPortsSameDT=off  OutDataTypeStr=boolean
  Test Airspeed : simulink/Logic and Bit Operations/Compare To Constant  relop=<  const=8  OutDataTypeStr=boolean
  Test Ground Spee : simulink/Logic and Bit Operations/Compare To Constant  relop=<  const=2  OutDataTypeStr=boolean
  gndSpd : Fcn  Expr=sqrt(u(1)^2 + u(2)^2)
  onGround : Outport
  wires:
  gndSpd/1 -> Test Ground Spee/1
  Test Airspeed/1 -> Logical Operator/2
  Test Ground Spee/1 -> Logical Operator/1
  Bus Selector/1 -> gndSpd/1  "<VelNED>"
  VtasMea/1 -> Test Airspeed/1
  Logical Operator/1 -> onGround/1
  PrepData/1 -> Bus Selector/1

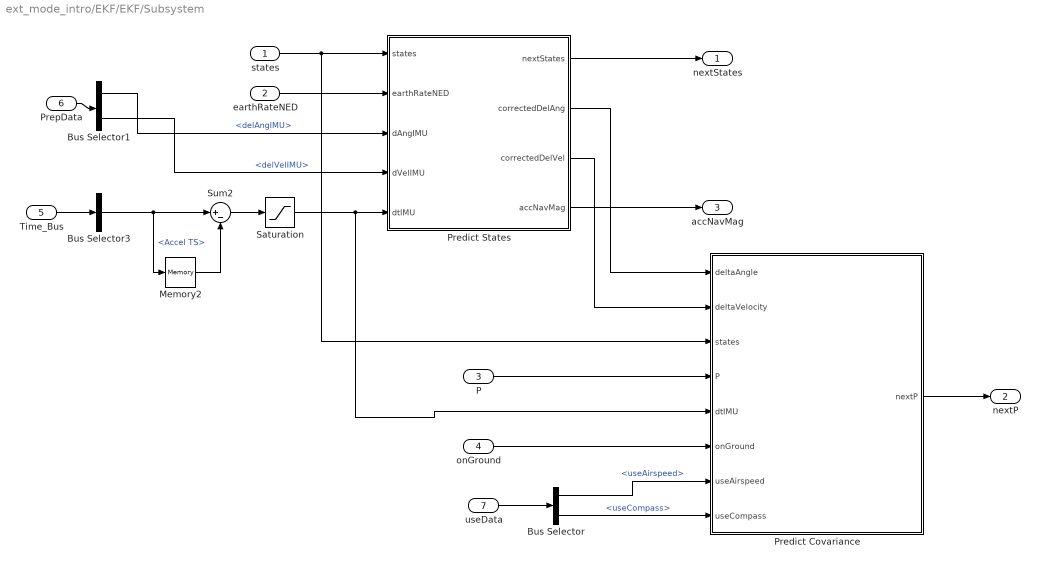
== system ext_mode_intro/EKF/EKF/Subsystem ==
  states : Inport
  earthRateNED : Inport  Port=2
  P : Inport  Port=3
  onGround : Inport  Port=4
  Time_Bus : Inport  Port=5
  PrepData : Inport  Port=6
  useData : Inport  Port=7
  Bus Selector : BusSelector  OutputSignals=useAirspeed,useCompass
  Bus Selector1 : BusSelector  OutputSignals=delAngIMU,delVelIMU
  Bus Selector3 : BusSelector  OutputSignals=Accel TS
  Memory2 : Memory  InheritSampleTime=on
  Predict Covariance : MATLAB Function  TreatAsAtomicUnit=on
  Predict States : MATLAB Function  TreatAsAtomicUnit=on
  Saturation : Saturate  UpperLimit=0.04  LowerLimit=0
  Sum2 : Sum  Inputs=|+-  AccumDataTypeStr=single
  nextStates : Outport
  nextP : Outport  Port=2
  accNavMag : Outport  Port=3
  wires:
  earthRateNED/1 -> Predict States/2(earthRateNED)
  states/1 -> Predict Covariance/3(states), Predict States/1(states)
  Predict States/4(accNavMag) -> accNavMag/1
  Bus Selector1/2 -> Predict States/4(dVelIMU)  "<delVelIMU>"
  Bus Selector1/1 -> Predict States/3(dAngIMU)  "<delAngIMU>"
  P/1 -> Predict Covariance/4(P)
  onGround/1 -> Predict Covariance/6(onGround)
  Predict States/2(correctedDelAng) -> Predict Covariance/1(deltaAngle)
  Predict States/1(nextStates) -> nextStates/1
  Predict States/3(correctedDelVel) -> Predict Covariance/2(deltaVelocity)
  Predict Covariance/1(nextP) -> nextP/1
  useData/1 -> Bus Selector/1
  Bus Selector/1 -> Predict Covariance/7(useAirspeed)  "<useAirspeed>"
  Bus Selector/2 -> Predict Covariance/8(useCompass)  "<useCompass>"
  Bus Selector3/1 -> Memory2/1, Sum2/1  "<Accel TS>"
  Memory2/1 -> Sum2/2
  Sum2/1 -> Saturation/1
  Time_Bus/1 -> Bus Selector3/1
  Saturation/1 -> Predict Covariance/5(dtIMU), Predict States/5(dtIMU)
  PrepData/1 -> Bus Selector1/1

== system ext_mode_intro/EKF/WatchDog/Get AHRS Data ==
  Angles : Inport
  Temp Angles : Inport  Port=2
  Demux : Demux  Outputs=3
  Mux5 : Mux  Inputs=3
  Terminator : Terminator
  wrapAng to +-pi : Subsystem
  Out1 : Outport
  wires:
  Demux/1 -> Mux5/1
  Demux/2 -> Mux5/2
  Demux/3 -> wrapAng to +-pi/1(In1)
  wrapAng to +-pi/1(Out1) -> Mux5/3
  Angles/1 -> Terminator/1
  Mux5/1 -> Out1/1
  Temp Angles/1 -> Demux/1

== system ext_mode_intro/EKF/WatchDog/Quat2Eul ==
  q : Inport  PortDimensions=4
  Mux : Mux  Inputs=3
  phi : Fcn  Expr=atan2(2*(u[3]*u[4]+u[1]*u[2] ) , u[1]^2-u[2]^2-u[3]^2+u[4]^2)
  psi : Fcn  Expr=atan2(2*(u[2]*u[3]+u[1]*u[4] ) , u[1]^2+u[2]^2-u[3]^2-u[4]^2)
  theta : Fcn  Expr=-asin(2*(u[2]*u[4]-u[1]*u[3]))
  Eul : Outport
  wires:
  Mux/1 -> Eul/1
  phi/1 -> Mux/1
  theta/1 -> Mux/2
  q/1 -> phi/1, theta/1, psi/1
  psi/1 -> Mux/3

== system ext_mode_intro/EKF/EKF/Initialize/Calc Initial Parameters ==
  Sensor_Bus : Inport
  Enable : EnablePort
  Bus Selector8 : BusSelector  OutputSignals=Latitude
  Embedded MATLAB Function : MATLAB Function  TreatAsAtomicUnit=on
  covariance : Outport
  earthRateNED : Outport  Port=2  PortDimensions=3
  wires:
  Embedded MATLAB Function/2(covariance) -> covariance/1
  Embedded MATLAB Function/1(earthRateNED) -> earthRateNED/1
  Bus Selector8/1 -> Embedded MATLAB Function/1(latDeg)  "<Latitude>"
  Sensor_Bus/1 -> Bus Selector8/1

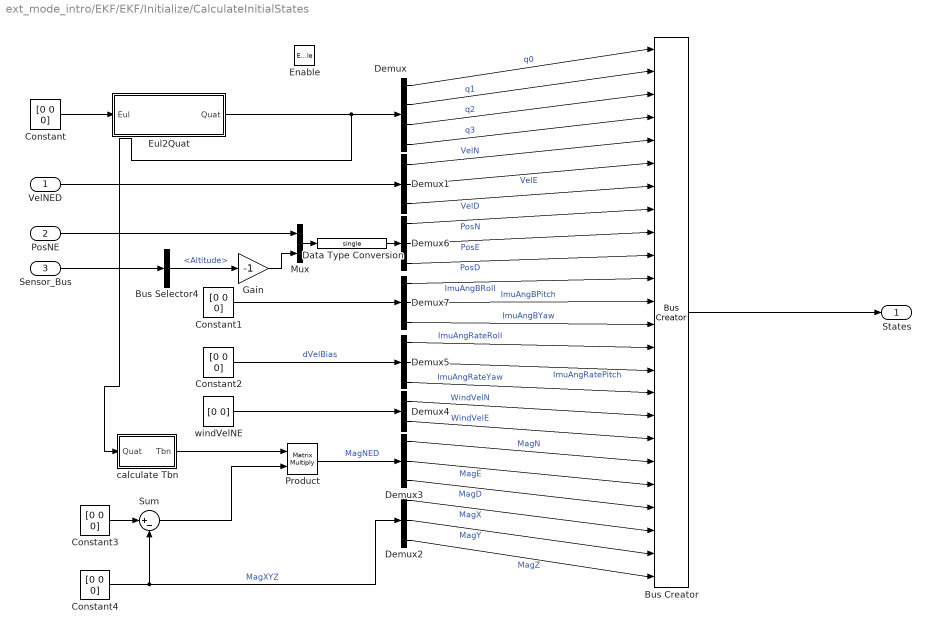
== system ext_mode_intro/EKF/EKF/Initialize/CalculateInitialStates ==
  VelNED : Inport  OutDataTypeStr=single
  PosNE : Inport  Port=2
  Sensor_Bus : Inport  Port=3
  Enable : EnablePort
  Bus Creator : BusCreator  Inputs=24
  Bus Selector4 : BusSelector  OutputSignals=Altitude
  Constant{,1..4} (5 alike) : Constant  Value=[0 0 0]  OutDataTypeStr=single  SampleTime=-1
  Data Type Conversion : DataTypeConversion  OutDataTypeStr=single
  Demux : Demux
  Demux{1..3,5..7} (6 alike) : Demux  Outputs=3
  Demux4 : Demux  Outputs=2
  Eul2Quat : Subsystem
  Gain : Gain  Gain=-1
  Mux : Mux  Inputs=2
  Product : Product  Multiplication=Matrix(*)  RndMeth=Zero
  Sum : Sum  Inputs=|+-
  calculate Tbn : Subsystem
  windVelNE : Constant  Value=[0 0]  OutDataTypeStr=single  SampleTime=-1
  States : Outport
  wires:
  Sum/1 -> Product/2
  Eul2Quat/1(Quat) -> calculate Tbn/1(Quat), Demux/1
  Bus Creator/1 -> States/1
  windVelNE/1 -> Demux4/1
  Constant2/1 -> Demux5/1  "dVelBias"
  VelNED/1 -> Demux1/1
  Gain/1 -> Mux/2
  PosNE/1 -> Mux/1
  Constant1/1 -> Demux7/1
  Bus Selector4/1 -> Gain/1  "<Altitude>"
  Constant/1 -> Eul2Quat/1(Eul)
  Constant3/1 -> Sum/1
  Constant4/1 -> Demux2/1, Sum/2  "MagXYZ"
  calculate Tbn/1(Tbn) -> Product/1
  Sensor_Bus/1 -> Bus Selector4/1
  Demux/1 -> Bus Creator/1  "q0"
  Demux/2 -> Bus Creator/2  "q1"
  Demux/3 -> Bus Creator/3  "q2"
  Demux/4 -> Bus Creator/4  "q3"
  Demux1/1 -> Bus Creator/5  "VelN"
  Demux1/2 -> Bus Creator/6  "VelE"
  Demux1/3 -> Bus Creator/7  "VelD"
  Demux2/3 -> Bus Creator/24  "MagZ"
  Demux2/2 -> Bus Creator/23  "MagY"
  Demux2/1 -> Bus Creator/22  "MagX"
  Demux3/1 -> Bus Creator/19  "MagN"
  Demux3/2 -> Bus Creator/20  "MagE"
  Demux3/3 -> Bus Creator/21  "MagD"
  Product/1 -> Demux3/1  "MagNED"
  Demux4/2 -> Bus Creator/18  "WindVelE"
  Demux4/1 -> Bus Creator/17  "WindVelN"
  Demux5/3 -> Bus Creator/16  "ImuAngRateYaw"
  Demux5/2 -> Bus Creator/15  "ImuAngRatePitch"
  Demux5/1 -> Bus Creator/14  "ImuAngRateRoll"
  Demux6/1 -> Bus Creator/8  "PosN"
  Demux6/2 -> Bus Creator/9  "PosE"
  Demux6/3 -> Bus Creator/10  "PosD"
  Demux7/1 -> Bus Creator/11  "ImuAngBRoll"
  Demux7/2 -> Bus Creator/12  "ImuAngBPitch"
  Demux7/3 -> Bus Creator/13  "ImuAngBYaw"
  Mux/1 -> Data Type Conversion/1
  Data Type Conversion/1 -> Demux6/1

== system ext_mode_intro/EKF/WatchDog/Get AHRS Data/wrapAng to +-pi ==
  In1 : Inport  OutDataTypeStr=single
  If : If  IfExpression=u1 > single(pi)
  If Action Subsystem : Subsystem  TreatAsAtomicUnit=on
  If Action Subsystem1 : Subsystem  TreatAsAtomicUnit=on
  Merge : Merge
  Out1 : Outport  OutDataTypeStr=single
  wires:
  In1/1 -> If Action Subsystem1/1(In1), If Action Subsystem/1(In1), If/1
  If/2 -> If Action Subsystem/Action
  If/1 -> If Action Subsystem1/Action
  If Action Subsystem/1(Out1) -> Merge/1
  If Action Subsystem1/1(Out1) -> Merge/2
  Merge/1 -> Out1/1

== system ext_mode_intro/EKF/EKF/Initialize/CalculateInitialStates/Eul2Quat ==
  Eul : Inport
  Gain : Gain  Gain=0.5  SaturateOnIntegerOverflow=on  OutDataTypeStr=Inherit: Same as input  ParamDataTypeStr=Inherit: Same as input
  Mux : Mux
  Mux1 : Mux  Inputs=[3 3]
  cos(0.5*E) : Trigonometry  Operator=cos
  q0 : Fcn  Expr=u[1] * u[2] * u[3] + u[4] * u[5] * u[6]
  q1 : Fcn  Expr=u[4] * u[2] * u[3] - u[1] * u[5] * u[6]
  q2 : Fcn  Expr=u[1] * u[5] * u[3] + u[4] * u[2] * u[6]
  q3 : Fcn  Expr=u[1] * u[2] * u[6] - u[4] * u[5] * u[3]
  sin(0.5*E)1 : Trigonometry
  Quat : Outport
  wires:
  Eul/1 -> Gain/1
  Gain/1 -> cos(0.5*E)/1, sin(0.5*E)1/1
  cos(0.5*E)/1 -> Mux1/1
  sin(0.5*E)1/1 -> Mux1/2
  q0/1 -> Mux/1
  Mux/1 -> Quat/1
  q1/1 -> Mux/2
  q2/1 -> Mux/3
  q3/1 -> Mux/4
  Mux1/1 -> q0/1, q1/1, q3/1, q2/1

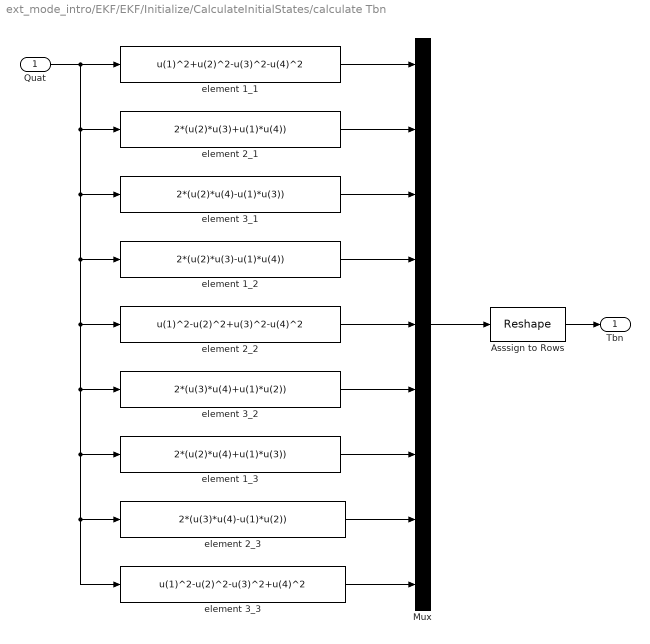
== system ext_mode_intro/EKF/EKF/Initialize/CalculateInitialStates/calculate Tbn ==
  Quat : Inport  PortDimensions=4
  Asssign to Rows : Reshape  OutputDimensionality=Customize  OutputDimensions=[3,3]
  Mux : Mux  Inputs=9
  element 1_1 : Fcn  Expr=u(1)^2+u(2)^2-u(3)^2-u(4)^2
  element 1_2 : Fcn  Expr=2*(u(2)*u(3)-u(1)*u(4))
  element 1_3 : Fcn  Expr=2*(u(2)*u(4)+u(1)*u(3))
  element 2_1 : Fcn  Expr=2*(u(2)*u(3)+u(1)*u(4))
  element 2_2 : Fcn  Expr=u(1)^2-u(2)^2+u(3)^2-u(4)^2
  element 2_3 : Fcn  Expr=2*(u(3)*u(4)-u(1)*u(2))
  element 3_1 : Fcn  Expr=2*(u(2)*u(4)-u(1)*u(3))
  element 3_2 : Fcn  Expr=2*(u(3)*u(4)+u(1)*u(2))
  element 3_3 : Fcn  Expr=u(1)^2-u(2)^2-u(3)^2+u(4)^2
  Tbn : Outport
  wires:
  Mux/1 -> Asssign to Rows/1
  element 1_1/1 -> Mux/1
  element 2_1/1 -> Mux/2
  element 3_1/1 -> Mux/3
  element 1_2/1 -> Mux/4
  element 2_2/1 -> Mux/5
  element 3_2/1 -> Mux/6
  element 1_3/1 -> Mux/7
  element 2_3/1 -> Mux/8
  element 3_3/1 -> Mux/9
  Asssign to Rows/1 -> Tbn/1
  Quat/1 -> element 1_1/1, element 3_3/1, element 2_3/1, element 1_3/1, element 3_2/1, element 2_2/1, element 1_2/1, element 3_1/1, element 2_1/1

== system ext_mode_intro/EKF/WatchDog/Get AHRS Data/wrapAng to +-pi/If Action Subsystem ==
  In1 : Inport
  Action Port : ActionPort  ActionType=else
  Out1 : Outport
  wires:
  In1/1 -> Out1/1

== system ext_mode_intro/EKF/WatchDog/Get AHRS Data/wrapAng to +-pi/If Action Subsystem1 ==
  In1 : Inport
  Action Port : ActionPort  ActionType=then
  Add : Sum  Inputs=+-
  Constant : Constant  Value=2*pi  OutDataTypeStr=single
  Out1 : Outport
  wires:
  In1/1 -> Add/1
  Add/1 -> Out1/1
  Constant/1 -> Add/2

== matlab function ext_mode_intro/EKF/EKF/Subsystem/Predict States ==
  data: nextStates output; correctedDelAng output; correctedDelVel output; accNavMag output; states input; earthRateNED input; dAngIMU input; dVelIMU input; dtIMU input
%#codegen
function [nextStates,correctedDelAng,correctedDelVel,accNavMag]  = UpdateStrapdownEquationsNED( ...
    states, ...
    earthRateNED, ...
    dAngIMU, ...
    dVelIMU, ...
    dtIMU)

% define persistent variables for previous delta angle and velocity which
% are required for sculling and coning error corrections
persistent prevDelAng;
if isempty(prevDelAng)
    prevDelAng = single([0;0;0]);
end
persistent Tbn;
if isempty(Tbn)
    Tbn = single(eye(3));
end

gravityNED = [0.0;0.0;9.80665];

% Remove sensor bias errors
correctedDelAng = dAngIMU - states(11:13);
correctedDelVel = dVelIMU - states(14:16);

% Save current measurements
prevDelAng = correctedDelAng;

% Apply corrections for earths rotation rate and coning errors
correctedDelAng   = correctedDelAng - transpose(Tbn)*earthRateNED*dtIMU + 8.333333333333333e-2*cross(prevDelAng , dAngIMU);

% Initialise the updated state vector
nextStates   = states;

% Convert the rotation vector to its equivalent quaternion
rotationMag = sqrt(correctedDelAng(1)^2 + correctedDelAng(2)^2 + correctedDelAng(3)^2);
if rotationMag<1e-12
  deltaQuat = single([1;0;0;0]);
else
  deltaQuat = [cos(0.5*rotationMag); correctedDelAng/rotationMag*sin(0.5*rotationMag)];
end

% Update the quaternions by rotating from the previous attitude through
% the delta angle rotation quaternion
qUpdated = [states(1)*deltaQuat(1)-transpose(states(2:4))*deltaQuat(2:4); states(1)*deltaQuat(2:4) + deltaQuat(1)*states(2:4) + cross(states(2:4),deltaQuat(2:4))];

% Normalise the quaternions and update the quaternion states
quatMag = sqrt(qUpdated(1)^2 + qUpdated(2)^2 + qUpdated(3)^2 + qUpdated(4)^2);
if (quatMag < 1e-16)
    nextStates(1:4) = qUpdated;
else
    nextStates(1:4) = qUpdated / quatMag;
end

% Calculate the body to nav cosine matrix
Tbn = [nextStates(1)^2 + nextStates(2)^2 - nextStates(3)^2 - nextStates(4)^2, 2*(nextStates(2)*nextStates(3) - nextStates(1)*nextStates(4)), 2*(nextStates(2)*nextStates(4) + nextStates(1)*nextStates(3));...
      2*(nextStates(2)*nextStates(3) + nextStates(1)*nextStates(4)), nextStates(1)^2 - nextStates(2)^2 + nextStates(3)^2 - nextStates(4)^2, 2*(nextStates(3)*nextStates(4) - nextStates(1)*nextStates(2));...
      2*(nextStates(2)*nextStates(4)-nextStates(1)*nextStates(3)), 2*(nextStates(3)*nextStates(4) + nextStates(1)*nextStates(2)), nextStates(1)^2 - nextStates(2)^2 - nextStates(3)^2 + nextStates(4)^2];
  
% transform body delta velocities to delta velocities in the nav frame
delVelNav = Tbn * correctedDelVel + gravityNED*dtIMU;

% calculate the magnitude of the nav acceleration (required for GPS
% variance estimation)
accNavMag = sqrt(delVelNav(1)^2 + delVelNav(2)^2 + delVelNav(3)^2) / dtIMU;

% If calculating position save previous velocity
lastVelocity = nextStates(5:7);

% Sum delta velocities to get velocity after removing gravitational skew and correcting for transport rate
nextStates(5:7) = states(5:7) + delVelNav;


% If calculating postions, do a trapezoidal integration for position
nextStates(8:10)     = states(8:10) + 0.5*(nextStates(5:7) + lastVelocity)*dtIMU;

% Copy the remaining states across
nextStates(11:24) = states(11:24);

end

== matlab function ext_mode_intro/EKF/EKF/Initialize/Calc Initial Parameters/Embedded MATLAB Function ==
  data: earthRateNED output; covariance output; latDeg input
function [earthRateNED, covariance] = calculateInitialData(latDeg)
%#codegen

% degrees to to radians conversion
deg2rad = single(pi/180);

% Define the initial Euler angle covariance (Phi, Theta, Psi)
InitialEulerCovariance  = single([(1.0*pi/180); (1.0*pi/180); (10.0*pi/180)].^2);

% Define the transformation vector from a 321 sequence Euler rotation vector to a q0,...,q3 quaternion vector
% linearised around a level orientation (roll,pitch = 0,0)
J_eul2quat = ...
    single([[ 0.0, 0.0, 0.0]; ...
    [ 0.5, 0.0, 0.0]; ...
    [ 0.0, 0.5, 0.0]; ...
    [ 0.0, 0.0, 0.5]]);

% Form the covariance matrix for the intial Euler angle coordinates
angleCov = diag(InitialEulerCovariance);

% Transform the Euler angle covariances into the equivalent quaternion covariances
quatCov = J_eul2quat*angleCov*transpose(J_eul2quat);

% define the state covariances with the exception of the quaternion covariances
Sigma_vel_NE = single(0.7); % 1 sigma uncertainty in horizontal velocity components
Sigma_vel_D  = single(0.7); % 1 sigma uncertainty in vertical velocity
Sigma_pos_NE = single(15); % 1 sigma uncertainty in horizontal position components
Sigma_pos_D  = single(5.0); % 1 sigma uncertainty in vertical position
Sigma_dAng   = single(1/10*pi/180*0.02); % 1 Sigma uncertainty in delta angle bias
Sigma_dVel   = single(0.1*0.02); % 1 Sigma uncertainty in delta velocity bias
Sigma_wind   = single(8);
Sigma_MagNED = single(20);
Sigma_MagXYZ = single(20);
covariance   = single(diag([0;0;0;0;Sigma_vel_NE*[1;1];Sigma_vel_D;Sigma_pos_NE*[1;1];Sigma_pos_D;Sigma_dAng*[1;1;1];Sigma_dVel*[1;1;1];Sigma_wind*[1;1];Sigma_MagNED*[1;1;1];Sigma_MagXYZ*[1;1;1]].^2));

% Add the quaternion covariances
covariance(1:4,1:4) = quatCov;

%Define Earth rotation vector in the NED navigation frame
earthRateECEF = single([0; 0; 7.2921e-005]);
earthRateNED  = ...
    single([cos(latDeg*deg2rad)*earthRateECEF(3); ...
    0; ...
    -sin(latDeg*deg2rad)*earthRateECEF(3)]);
